simulink model "ex7_4"  (R2015a)
settings: Solver=ode23t  SolverMode=SingleTasking  StartTime=0.0  StopTime=.3  MaxStep=1e-5  RelTol=1e-3
libraries: powerlib x17, powerlib_meascontrol x4, simulink x2
settings Model: CovMetricSettings=dwe  CovHtmlReporting=off  covSaveCumulativeToWorkspaceVar=off  CovSaveSingleToWorkspaceVar=off  CovExternalEMLEnable=on  Creator=Omid  LastModifiedBy=Omid
settings SolverCC: ZeroCrossAlgorithm=Adaptive
settings DataIOCC: LimitDataPoints=off  SaveFormat=Dataset  ReturnWorkspaceOutputs=on
settings DebuggingCC: IgnoredZcDiagnostic=none  UnconnectedInputMsg=none  UnconnectedOutputMsg=none  UnconnectedLineMsg=none  SFUnexpectedBacktrackingDiag=error  SFNoUnconditionalDefaultTransitionDiag=error
settings HardwareCC: ProdBitPerPointer=64  ProdLargestAtomicFloat=Float  ProdIntDivRoundTo=Zero  ProdEndianess=LittleEndian  ProdHWDeviceType=Specified
settings ModelReferenceCC: PropagateSignalLabelsOutOfModel=on
settings SFSimCC: SimUseLocalCustomCode=on
settings RTWCC: RTWUseLocalCustomCode=on
settings GRTTargetCC: TargetLangStandard=C99 (ISO)
settings ConfigurationSet: Description=Simscape Multibody

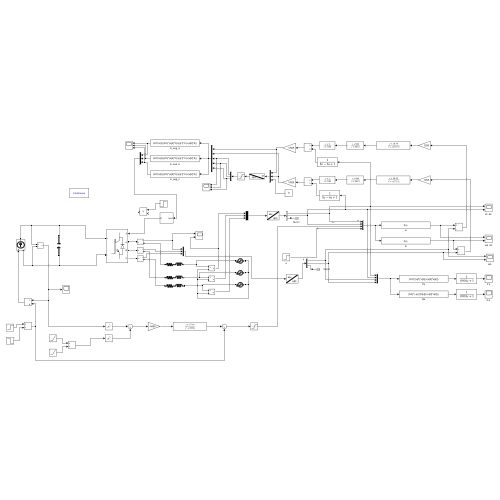
[thumbnail: Simulink's stored preview of the top-level diagram]
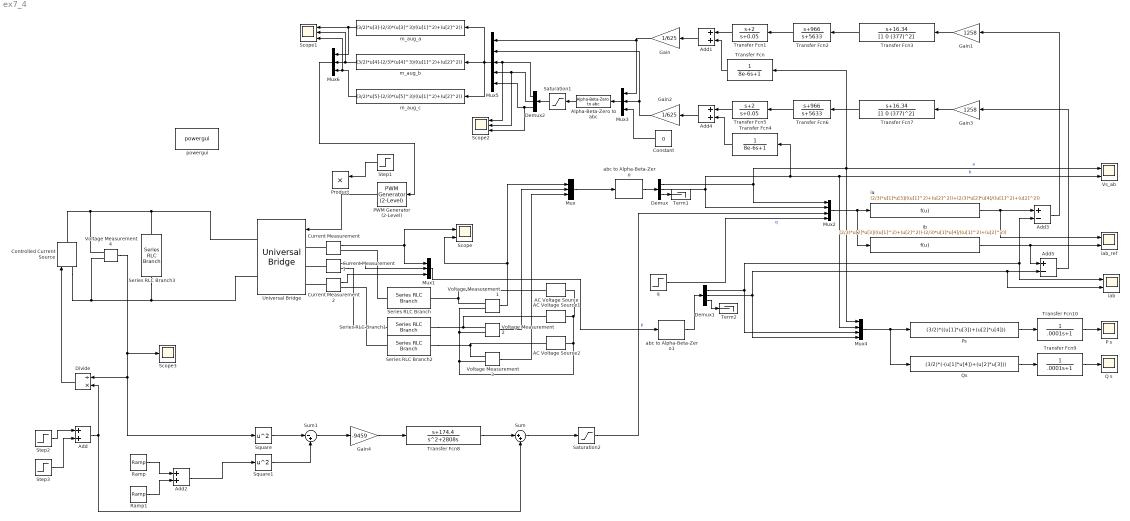
== system ex7_4 ==
  AC Voltage Source : powerlib/Electrical Sources/AC Voltage Source  Amplitude=391  Phase=0  Frequency=60  SampleTime=0  Measurements=None  BusType=swing  Pref=10e3  Qref=0  Qmin=-inf  Qmax=+inf
  AC Voltage Source1 : powerlib/Electrical Sources/AC Voltage Source  Amplitude=391  Phase=120  Frequency=60  SampleTime=0  Measurements=None  BusType=swing  Pref=10e3  Qref=0  Qmin=-inf  Qmax=+inf
  AC Voltage Source2 : powerlib/Electrical Sources/AC Voltage Source  Amplitude=391  Phase=240  Frequency=60  SampleTime=0  Measurements=None  BusType=swing  Pref=10e3  Qref=0  Qmin=-inf  Qmax=+inf
  Add{,1..2,4} (4 alike) : Sum
  Add3 : Sum  Inputs=+-
  Add5 : Sum  Inputs=+-
  Alpha-Beta-Zero to abc : powerlib_meascontrol/Transformations/Alpha-Beta-Zero to abc
  Constant : Constant  Value=0
  Controlled Current Source : powerlib/Electrical Sources/Controlled Current Source  Initialize=on  Source_Type=DC  Amplitude=0  Phase=0  Frequency=0  Measurements=None
  Current Measurement : powerlib/Measurements/Current Measurement  PhasorSimulation=off  OutputType=Complex  PSBequivalent=0
  Current Measurement1 : powerlib/Measurements/Current Measurement  PhasorSimulation=off  OutputType=Complex  PSBequivalent=0
  Current Measurement2 : powerlib/Measurements/Current Measurement  PhasorSimulation=off  OutputType=Complex  PSBequivalent=0
  Demux : Demux  Outputs=3
      settings: DisplayOption=none
  Demux1 : Demux  Outputs=3
  Demux2 : Demux  Outputs=3
  Divide : Product  Inputs=/*
  Gain : Gain  Gain=1/625
  Gain1 : Gain  Gain=1258
  Gain2 : Gain  Gain=1/625
  Gain3 : Gain  Gain=1258
  Gain4 : Gain  Gain=-9459
  Mux{,1,3,6} (4 alike) : Mux  Inputs=3
  Mux2 : Mux
  Mux4 : Mux
  Mux5 : Mux  Inputs=5
  P s : Scope
      settings: TimeRange=auto  MaxDataPoints=5000  SaveToWorkspace=off  SaveName=ScopeData4  YMin=-2749945.63227  YMax=1784575.09164  SampleTime=-1
  PWM Generator (2-Level) : powerlib_meascontrol/Pulse & Signal Generators/PWM Generator (2-Level)  ModulatorType=Three-phase bridge (6 pulses)  ModulatorMode=Unsynchronized  Fc=3420  Pc=90  nF=27  MinMax="[ -1  1 ]"  SamplingTechnique=Natural  ModulatingSignals=off  m=0.8  Freq=60  Phase=0  Ts=0  ShowCarrierOutport=off
  Product : Product
  Ps : Fcn  Expr=(3/2)*((u[1]*u[3])+(u[2]*u[4]))
  Q s : Scope
      settings: TimeRange=auto  MaxDataPoints=5000  SaveToWorkspace=off  SaveName=ScopeData5  YMin=-493389.72463  YMax=856699.45372  SampleTime=-1
  Qs : Fcn  Expr=(3/2)*(-(u[1]*u[4])+(u[2]*u[3]))
  Ramp : simulink/Sources/Ramp  slope=50000  start=0  X0=660
  Ramp1 : simulink/Sources/Ramp  slope=-50000  start=.0118  X0=0
  Saturation1 : Saturate  UpperLimit=1  LowerLimit=-1
  Saturation2 : Saturate  UpperLimit=3.5e6  LowerLimit=-3.5e6
  Scope : Scope  NumInputPorts=2
      settings: TimeRange=auto  MaxDataPoints=5000  SaveToWorkspace=off  SaveName=ScopeData  YMin=-6000~-5  YMax=6000~5  SampleTime=-1
  Scope1 : Scope  NumInputPorts=3
      settings: TimeRange=auto  MaxDataPoints=5000  SaveToWorkspace=off  YMin=-0.99689~-5~-5  YMax=1.1913~5~5  SampleTime=-1
  Scope2 : Scope  NumInputPorts=3
      settings: TimeRange=auto  MaxDataPoints=5000  SaveToWorkspace=off  SaveName=ScopeData2  YMin=-1.24031~-5~-5  YMax=1.16279~5~5  SampleTime=-1
  Scope3 : Scope
      settings: TimeRange=auto  MaxDataPoints=5000  SaveToWorkspace=off  SaveName=ScopeData3  YMin=573.46764  YMax=1437.95493  SampleTime=-1
  Series RLC Branch : powerlib/Elements/Series RLC Branch  LConnTagsString=__new0  RConnTagsString=__new0  BranchType=RL  Resistance=.00075  Inductance=100e-6  SetiL0=off  InitialCurrent=1600  Capacitance=1e-6  Setx0=off  InitialVoltage=0  Measurements=None
  Series RLC Branch1 : powerlib/Elements/Series RLC Branch  LConnTagsString=__new0  RConnTagsString=__new0  BranchType=RL  Resistance=.00075  Inductance=100e-6  SetiL0=off  InitialCurrent=1600  Capacitance=1e-6  Setx0=off  InitialVoltage=0  Measurements=None
  Series RLC Branch2 : powerlib/Elements/Series RLC Branch  LConnTagsString=__new0  RConnTagsString=__new0  BranchType=RL  Resistance=.00075  Inductance=100e-6  SetiL0=off  InitialCurrent=1600  Capacitance=1e-6  Setx0=off  InitialVoltage=0  Measurements=None
  Series RLC Branch3 : powerlib/Elements/Series RLC Branch  LConnTagsString=__new0  RConnTagsString=__new0  BranchType=C  Resistance=1  Inductance=1e-3  SetiL0=off  InitialCurrent=0  Capacitance=9625e-6  Setx0=on  InitialVoltage=660  Measurements=None
  Square : Math  Operator=square  SaturateOnIntegerOverflow=on
  Square1 : Math  Operator=square  SaturateOnIntegerOverflow=on
  Step1 : Step  Time=.1  SampleTime=0
  Step2 : Step  Time=.1372  After=1e6  SampleTime=0
  Step3 : Step  Time=.2  After=-2e6  SampleTime=0
  Sum : Sum  Inputs=|++
  Sum1 : Sum  Inputs=|-+
  Term1 : Terminator
  Term2 : Terminator
  Transfer Fcn : TransferFcn  Denominator=[8e-6 1]
  Transfer Fcn1 : TransferFcn  Numerator=[1 2]  Denominator=[1 0.05]
  Transfer Fcn10 : TransferFcn  Denominator=[.0001 1]
  Transfer Fcn2 : TransferFcn  Numerator=[1 966]  Denominator=[1 5633]
  Transfer Fcn3 : TransferFcn  Numerator=[1 16.34]  Denominator=[1 0 (377)^2]
  Transfer Fcn4 : TransferFcn  Denominator=[8e-6 1]
  Transfer Fcn5 : TransferFcn  Numerator=[1 2]  Denominator=[1 0.05]
  Transfer Fcn6 : TransferFcn  Numerator=[1 966]  Denominator=[1 5633]
  Transfer Fcn7 : TransferFcn  Numerator=[1 16.34]  Denominator=[1 0 (377)^2]
  Transfer Fcn8 : TransferFcn  Numerator=[1 174.4]  Denominator=[1 2808 0]
  Transfer Fcn9 : TransferFcn  Denominator=[.0001 1]
  Universal Bridge : powerlib/Power Electronics/Universal Bridge  Arms=3  SnubberResistance=1e5  SnubberCapacitance=inf  Device=IGBT / Diodes  Ron=.88e-3  Lon=0  ForwardVoltages="[  1  1 ]"  ForwardVoltage=0  GTOparameters=[ 10e-6 , 20e-6 ]  IGBTparameters=[ 1e-6 , 2e-6 ]  Measurements=None  Measurements_2=None  converterType=Rectifier
  Voltage Measurement{1..4} (4 alike) : powerlib/Measurements/Voltage Measurement  PhasorSimulation=off  OutputType=Complex  PSBequivalent=0
  "Vs_ab " : Scope  NumInputPorts=2
      settings: TimeRange=auto  MaxDataPoints=5000  SaveToWorkspace=off  SaveName=ScopeData3  YMin=-2483.2971~-5  YMax=2875.43543~5  SampleTime=-1
  abc to Alpha-Beta-Zero : powerlib_meascontrol/Transformations/abc to Alpha-Beta-Zero
  abc to Alpha-Beta-Zero1 : powerlib_meascontrol/Transformations/abc to Alpha-Beta-Zero
  ia : Fcn  Expr=(2/3)*u[1]*u[3]/((u[1]^2)+(u[2]^2))+(2/3)*u[2]*u[4]/((u[1]^2)+(u[2]^2))
  iab : Scope  NumInputPorts=2
      settings: TimeRange=auto  MaxDataPoints=5000  SaveToWorkspace=off  SaveName=ScopeData2  YMin=-2627.79155~-5  YMax=2833.00726~5  SampleTime=-1
  iab_ref : Scope  NumInputPorts=2
      settings: TimeRange=auto  MaxDataPoints=5000  SaveToWorkspace=off  YMin=-6000~-5  YMax=6000~5  SampleTime=-1
  ib : Fcn  Expr=(2/3)*u[2]*u[3]/((u[1]^2)+(u[2]^2))-(2/3)*u[1]*u[4]/((u[1]^2)+(u[2]^2))
  m_aug_a : Fcn  Expr=(3/2)*u[3]-(2/3)*(u[3]^3)/((u[1]^2)+(u[2]^2))
  m_aug_b : Fcn  Expr=(3/2)*u[4]-(2/3)*(u[4]^3)/((u[1]^2)+(u[2]^2))
  m_aug_c : Fcn  Expr=(3/2)*u[5]-(2/3)*(u[5]^3)/((u[1]^2)+(u[2]^2))
  powergui : powerlib/powergui  Priority=1  SimulationMode=Continuous  SampleTime=50e-6  frequency=60  Iterations=50  frequencyindice=0  Pbase=100e6  ErrMax=1e-4  UnitsV=kV  UnitsW=MW  buscounter=0  FunctionMessages=off  echomessages=off  EnableUseOfTLC=off  CurrentSourceSwitches=off  DisableSnubberDevices=off  DisableRonSwitches=off  DisableVfSwitches=off  DisplayEquations=off  AutomaticDiscreteSolvers=off  SolverType=Tustin/Backward Euler (TBE)  Interpol=off  ExternalGateDelay=off  methode=off  Ts=100  x0status=blocks  SPID=on  SwTol=0  HookPort=off  NonlinearTolerance=1e-4  nMaxIteration=100  ContinueOnMaxIteration=off  RestoreLinks=warning  ResistiveCurrentMeasurement=off  Frange=[0:2:500]  Ylog=off  Xlog=on  ShowGrid=off  save=off  variable=ZData  structure=0  ZoomFFT=off  StartTime=0.0  cycles=1  DisplayStyle=1  fundamental=60  FreqAxis=off  MaxFrequency=1000  frequencyindicesteady=1  RmsSteady=1  display=off
  q : Step  Time=.25  After=5e5  SampleTime=0
  wires:
  Add1/1 -> Gain/1
  Voltage Measurement1/1 -> Mux/1, Scope/2
  Transfer Fcn/1 -> Add1/2
  Transfer Fcn1/1 -> Add1/1
  Add3/1 -> Gain1/1
  Transfer Fcn2/1 -> Transfer Fcn1/1
  Transfer Fcn3/1 -> Transfer Fcn2/1
  Gain1/1 -> Transfer Fcn3/1
  Voltage Measurement3/1 -> Mux/3
  Voltage Measurement2/1 -> Mux/2
  Mux/1 -> abc to Alpha-Beta-Zero/1
  abc to Alpha-Beta-Zero/1 -> Demux/1
  abc to Alpha-Beta-Zero1/1 -> Demux1/1
  Mux1/1 -> abc to Alpha-Beta-Zero1/1
  Current Measurement1/1 -> Mux1/2
  Current Measurement2/1 -> Mux1/3
  Demux/1 -> Transfer Fcn/1, Mux4/1, "Vs_ab "/1, Mux2/1  "a"
  Demux/2 -> Transfer Fcn4/1, Mux4/2, "Vs_ab "/2, Mux2/2  "b"
  Saturation2/1 -> Mux2/3  "p"
  q/1 -> Mux2/4  "q"
  Mux2/1 -> ia/1, ib/1
  ia/1 -> Add3/1, iab_ref/1
  Demux1/1 -> iab/1, Add3/2, Mux4/3
  Gain3/1 -> Transfer Fcn7/1
  Transfer Fcn7/1 -> Transfer Fcn6/1
  Transfer Fcn6/1 -> Transfer Fcn5/1
  Transfer Fcn5/1 -> Add4/1
  Transfer Fcn4/1 -> Add4/2
  Add4/1 -> Gain2/1
  Add5/1 -> Gain3/1
  ib/1 -> iab_ref/2, Add5/1
  Demux1/2 -> iab/2, Add5/2, Mux4/4
  Alpha-Beta-Zero to abc/1 -> Saturation1/1
  Gain2/1 -> Mux3/2, Mux5/2
  Gain/1 -> Mux3/1, Mux5/1
  PWM Generator (2-Level)/1 -> Universal Bridge/1
  Mux3/1 -> Alpha-Beta-Zero to abc/1
  Constant/1 -> Mux3/3
  Current Measurement/1 -> Mux1/1, Scope/1
  Demux1/3 -> Term2/1
  Demux/3 -> Term1/1
  Mux4/1 -> Qs/1, Ps/1
  Demux2/1 -> Mux5/3, Scope2/1
  Demux2/2 -> Scope2/2, Mux5/4
  Demux2/3 -> Scope2/3, Mux5/5
  Mux5/1 -> m_aug_a/1, m_aug_b/1, m_aug_c/1
  m_aug_c/1 -> Scope1/3, Mux6/3
  Saturation1/1 -> Demux2/1
  Mux6/1 -> PWM Generator (2-Level)/1
  m_aug_a/1 -> Mux6/1, Scope1/1
  m_aug_b/1 -> Scope1/2, Mux6/2
  Gain4/1 -> Transfer Fcn8/1
  Sum/1 -> Saturation2/1
  Sum1/1 -> Gain4/1
  Square1/1 -> Sum1/2
  Step3/1 -> Add/2
  Step2/1 -> Add/1
  Voltage Measurement4/1 -> Scope3/1, Square/1, Divide/1
  Divide/1 -> Controlled Current Source/1
  Transfer Fcn8/1 -> Sum/1
  Step1/1 -> Product/1
  Add/1 -> Divide/2, Sum/2
  Ramp/1 -> Add2/1
  Ramp1/1 -> Add2/2
  Add2/1 -> Square1/1
  Square/1 -> Sum1/1
  Qs/1 -> Transfer Fcn9/1
  Transfer Fcn9/1 -> Q s/1
  Ps/1 -> Transfer Fcn10/1
  Transfer Fcn10/1 -> P s/1
  connections:
  Controlled Current Source/RConn1 -- Universal Bridge/RConn1 -- Series RLC Branch3/LConn1 -- Voltage Measurement4/LConn1
  Current Measurement/LConn1 -- Universal Bridge/LConn1
  Series RLC Branch/LConn1 -- Current Measurement/RConn1
  Voltage Measurement1/LConn1 -- AC Voltage Source/RConn1 -- Series RLC Branch/RConn1
  Current Measurement1/LConn1 -- Universal Bridge/LConn2
  Current Measurement1/RConn1 -- Series RLC Branch1/LConn1
  Voltage Measurement2/LConn1 -- Series RLC Branch1/RConn1 -- AC Voltage Source1/RConn1
  Current Measurement2/LConn1 -- Universal Bridge/LConn3
  Series RLC Branch2/LConn1 -- Current Measurement2/RConn1
  AC Voltage Source2/RConn1 -- Series RLC Branch2/RConn1 -- Voltage Measurement3/LConn1
  Controlled Current Source/LConn1 -- Voltage Measurement4/LConn2 -- Universal Bridge/RConn2 -- Series RLC Branch3/RConn1
  Voltage Measurement2/LConn2 -- AC Voltage Source/LConn1 -- AC Voltage Source1/LConn1 -- AC Voltage Source2/LConn1 -- Voltage Measurement3/LConn2 -- Voltage Measurement1/LConn2
